simulink subsystem "PowerSystemRef"  (R2024b)
settings: Solver=VariableStepAuto  StartTime=0.0  StopTime=10.0  RelTol=1e-3
undefined symbols (not defined in the file): ess, geom, mot, mot2, mot3, mot4, propel, propel2, propel3, propel4, pxf_diagram_options, SimIn, tc, tc2, tc3, tc4
libraries: simulink x10, slpidlib x5
(part 1 of 10)
settings Model: Creator=drhill  LastModifiedBy=John Clardy
settings SolverCC: AlgebraicLoopSolver=TrustRegion
settings OptimizationCC: ReuseModelBlockBuffer=off
settings DebuggingCC: UnconnectedInputMsg=warning  UnconnectedOutputMsg=warning  UnconnectedLineMsg=warning
settings ModelReferenceCC: EnableRefExpFcnMdlSchedulingChecks=on
settings RTWCC: GPUComputeCapability=3.5  DLArmComputeVersion=19.05

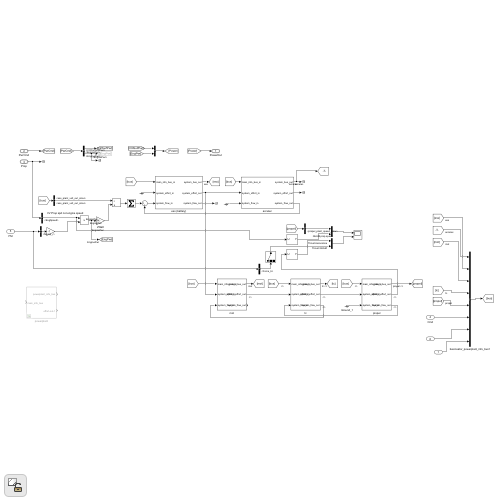
[thumbnail: Simulink's stored preview of the top-level diagram]
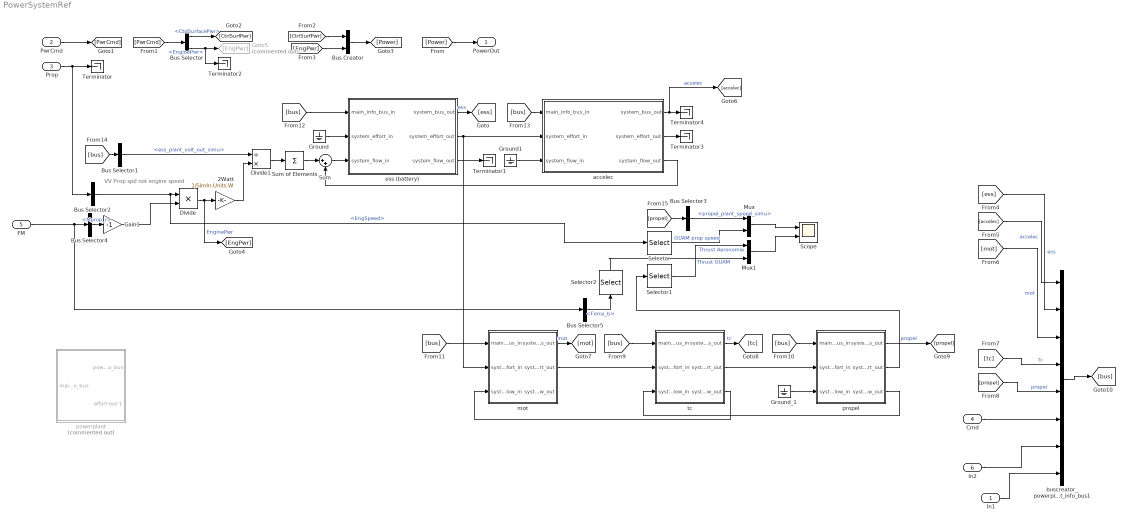
== system PowerSystemRef ==
  note: VV Prop spd not engine speed
  In1 : Inport
  PwrCmd : Inport  Port=2  OutDataTypeStr=Bus: BUS_POWER_SYSTEM_IN
  Prop : Inport  Port=3  OutDataTypeStr=Bus: BUS_PROP_ACTUATOR
  Cmd : Inport  Port=4
  FM : Inport  Port=5
  In2 : Inport  Port=6
  2Watt : Gain  Gain=1/SimIn.Units.W
  Bus Creator : BusCreator  Inputs=2  OutDataTypeStr=Bus: BUS_POWER_SYSTEM_OUT
  Bus Selector : BusSelector  OutputSignals=CtrlSurfacePwr,EnginePwr
  Bus Selector1 : BusSelector  OutputSignals=ess.plant.ess_plant_volt_out_simu
  Bus Selector2 : BusSelector  OutputSignals=EngSpeed
  Bus Selector3 : BusSelector  OutputSignals=propel_plant_speed_simu
  Bus Selector4 : BusSelector  OutputSignals=Propulsion.Mprop_r
  Bus Selector5 : BusSelector  OutputSignals=Propulsion.Force_b
  Divide : Product  Inputs=**
  Divide1 : Product  Inputs=/*
  Gain1 : Gain  Gain=-1
  Goto5 : Goto  Commented=on  GotoTag=EngPwr
  Ground : Ground
  Ground1 : Ground
  Ground_1 : Ground
  Mux : Mux  Inputs=2
  Mux1 : Mux  Inputs=2
  Scope : Scope  NumInputPorts=2
  Selector : Selector  InputPortWidth=9  IndexOptions=Index vector (dialog)  Indices=9  OutputSizes=1
  Selector1 : Selector  InputPortWidth=6  IndexOptions=Index vector (dialog)  Indices=1  OutputSizes=1
  Selector2 : Selector  InputPortWidth=3  IndexOptions=Index vector (dialog)  Indices=1  OutputSizes=1
  Sum : Sum  Inputs=|++
  Sum of Elements : Sum  Inputs=+
  Terminator{,1..4} (5 alike) : Terminator
  accelec : Subsystem
  buscreator_powerplant_info_bus1 : BusCreator  Inputs=8
  ess (battery) : Subsystem
  mot : Subsystem
  powerplant : Subsystem  Commented=on
  propel : Subsystem
  tc : Subsystem
  PowerOut : Outport  OutDataTypeStr=Bus: BUS_POWER_SYSTEM_OUT  VectorParamsAs1DForOutWhenUnconnected=off
  wires:
  Bus Creator/1 -> [Power]
  [Power] -> PowerOut/1
  PwrCmd/1 -> [PwrCmd]
  [PwrCmd] -> Bus Selector/1
  Bus Selector/1 -> [CtrlSurfPwr]  "<CtrlSurfacePwr>"
  [CtrlSurfPwr] -> Bus Creator/1
  [EngPwr] -> Bus Creator/2
  Ground/1 -> ess (battery)/2(system_effort_in)
  Bus Selector2/1 -> Divide/1, Selector/1  "<EngSpeed>"
  Divide1/1 -> Sum of Elements/1
  Prop/1 -> Terminator/1, Bus Selector2/1
  Divide/1 -> 2Watt/1, [EngPwr]  "EnginePwr"
  ess (battery)/3(system_flow_out) -> Terminator1/1
  Bus Selector1/1 -> Divide1/1  "<ess_plant_volt_out_simu>"
  Sum of Elements/1 -> Sum/1
  2Watt/1 -> Divide1/2
  Bus Selector4/1 -> Gain1/1  "<Mprop_r>"
  FM/1 -> Bus Selector4/1, Bus Selector5/1
  Gain1/1 -> Divide/2
  Bus Selector/2 -> Goto5/1, Terminator2/1  "<EnginePwr>"
  ess (battery)/2(system_effort_out) -> mot/2(system_effort_in), accelec/2(system_effort_in)
  Ground1/1 -> accelec/3(system_flow_in)
  Sum/1 -> ess (battery)/3(system_flow_in)
  accelec/3(system_flow_out) -> Sum/2
  accelec/2(system_effort_out) -> Terminator3/1
  accelec/1(system_bus_out) -> Terminator4/1, [accelec]  "accelec"
  [accelec] -> buscreator_powerplant_info_bus1/1  "accelec"
  [ess] -> buscreator_powerplant_info_bus1/2  "ess"
  [mot] -> buscreator_powerplant_info_bus1/3  "mot"
  mot/1(system_bus_out) -> [mot]  "mot"
  [tc] -> buscreator_powerplant_info_bus1/4  "tc"
  [propel] -> buscreator_powerplant_info_bus1/5  "propel"
  buscreator_powerplant_info_bus1/1 -> [bus]
  [bus] -> mot/1(main_info_bus_in)
  Cmd/1 -> buscreator_powerplant_info_bus1/6
  In1/1 -> buscreator_powerplant_info_bus1/8
  [bus] -> ess (battery)/1(main_info_bus_in)
  [bus] -> accelec/1(main_info_bus_in)
  ess (battery)/1(system_bus_out) -> [ess]  "ess"
  [bus] -> Bus Selector1/1
  In2/1 -> buscreator_powerplant_info_bus1/7
  Mux/1 -> Scope/1
  Mux1/1 -> Scope/2
  [propel] -> Bus Selector3/1
  Bus Selector3/1 -> Mux/1  "<propel_plant_speed_simu>"
  Selector/1 -> Mux/2  "GUAM prop speed"
  Selector1/1 -> Mux1/1  "Thrust Aeronomie"
  Bus Selector5/1 -> Selector2/1  "<Force_b>"
  Selector2/1 -> Mux1/2  "Thrust GUAM"
  mot/2(system_effort_out) -> tc/2(system_effort_in)
  tc/3(system_flow_out) -> mot/3(system_flow_in)
  tc/1(system_bus_out) -> [tc]  "tc"
  [bus] -> tc/1(main_info_bus_in)
  propel/2(system_effort_out) -> Selector1/1
  Ground_1/1 -> propel/3(system_flow_in)
  tc/2(system_effort_out) -> propel/2(system_effort_in)
  propel/3(system_flow_out) -> tc/3(system_flow_in)
  [bus] -> propel/1(main_info_bus_in)
  propel/1(system_bus_out) -> [propel]  "propel"

== system PowerSystemRef/accelec ==
  main_info_bus_in : Inport
  system_effort_in : Inport  Port=2
  system_flow_in : Inport  Port=3
  Ground_1 : Ground
  Terminator_1 : Terminator
  plant : Subsystem
      mask Display: disp('accelec_plant_const_pwrloss_volt_in_nokey.slx')
  system_bus_out : Outport
  system_effort_out : Outport  Port=2
  system_flow_out : Outport  Port=3
  wires:
  main_info_bus_in/1 -> plant/1(aInport--1)
  plant/1(outport-system_info_bus) -> [plant]
  plant/3(out-effort-6) -> system_effort_out/1
  plant/4(out-flow-7) -> system_flow_out/1
  system_effort_in/1 -> plant/3(in-effort-2)
  system_flow_in/1 -> plant/4(in-flow-3)
  [plant] -> system_bus_out/1  "plant"
  Ground_1/1 -> plant/2(aInport--2)
  plant/2(aOutport--2) -> Terminator_1/1

== system PowerSystemRef/ess (battery) ==
  main_info_bus_in : Inport
  system_effort_in : Inport  Port=2
  system_flow_in : Inport  Port=3
  buscreator_system_bus_out1 : BusCreator  Inputs=2
  ctrl : Subsystem
      mask Display: disp('ess_ctrl_pngv_map_anl_PI_cstr.slx')
  memoryctrl : Memory
  plant : Subsystem
      mask Display: disp('ess_plant_pngv_map_anl_PI_cstr.slx')
  system_bus_out : Outport
  system_effort_out : Outport  Port=2
  system_flow_out : Outport  Port=3
  wires:
  ctrl/1(outport-system_info_bus) -> [ctrl]  "system_info_bus"
  ctrl/2(outport-ctrl_bus) -> memoryctrl/1  "ctrl_bus"
  main_info_bus_in/1 -> ctrl/1(inport-main_info_bus-1), plant/1(aInport--1)  "main_info_bus"
  plant/2(outport-plant_bus) -> ctrl/2(aInport--2)  "plant_bus"
  memoryctrl/1 -> plant/2(aInport--2)  "ctrl_bus"
  plant/1(outport-system_info_bus) -> [plant]  "system_info_bus"
  plant/3(out-effort-12) -> system_effort_out/1  "effort"
  plant/4(out-flow-13) -> system_flow_out/1  "flow"
  system_effort_in/1 -> plant/3(in-effort-1)  "effort"
  system_flow_in/1 -> plant/4(in-flow-2)  "flow"
  buscreator_system_bus_out1/1 -> system_bus_out/1  "system_info_bus"
  [ctrl] -> buscreator_system_bus_out1/1  "ctrl"
  [plant] -> buscreator_system_bus_out1/2  "plant"

== system PowerSystemRef/mot ==
  main_info_bus_in : Inport
  system_effort_in : Inport  Port=2
  system_flow_in : Inport  Port=3
  buscreator_system_bus_out1 : BusCreator  Inputs=2
  ctrl : Subsystem
  memoryctrl : Memory
  plant : Subsystem
      mask Display: disp('mot_plant_map_Pelec_funTW_volt_in.slx')
  system_bus_out : Outport
  system_effort_out : Outport  Port=2
  system_flow_out : Outport  Port=3
  wires:
  ctrl/1(system_bus_out) -> [ctrl]  "system_info_bus"
  ctrl/2(local_info_bus_out) -> memoryctrl/1  "ctrl_bus"
  main_info_bus_in/1 -> ctrl/1(main_info_bus_in), plant/1(aInport--1)  "main_info_bus"
  plant/2(outport-plant_bus) -> ctrl/2(local_info_bus_in)  "plant_bus"
  memoryctrl/1 -> plant/2(inport-ctrl_bus-2)  "ctrl_bus"
  plant/1(outport-system_info_bus) -> [plant]  "system_info_bus"
  plant/3(out-effort-7) -> system_effort_out/1  "effort"
  plant/4(out-flow-8) -> system_flow_out/1  "flow"
  system_effort_in/1 -> plant/3(in-effort-2)  "effort"
  system_flow_in/1 -> plant/4(in-flow-3)  "flow"
  buscreator_system_bus_out1/1 -> system_bus_out/1  "system_info_bus"
  [ctrl] -> buscreator_system_bus_out1/1  "ctrl"
  [plant] -> buscreator_system_bus_out1/2  "plant"

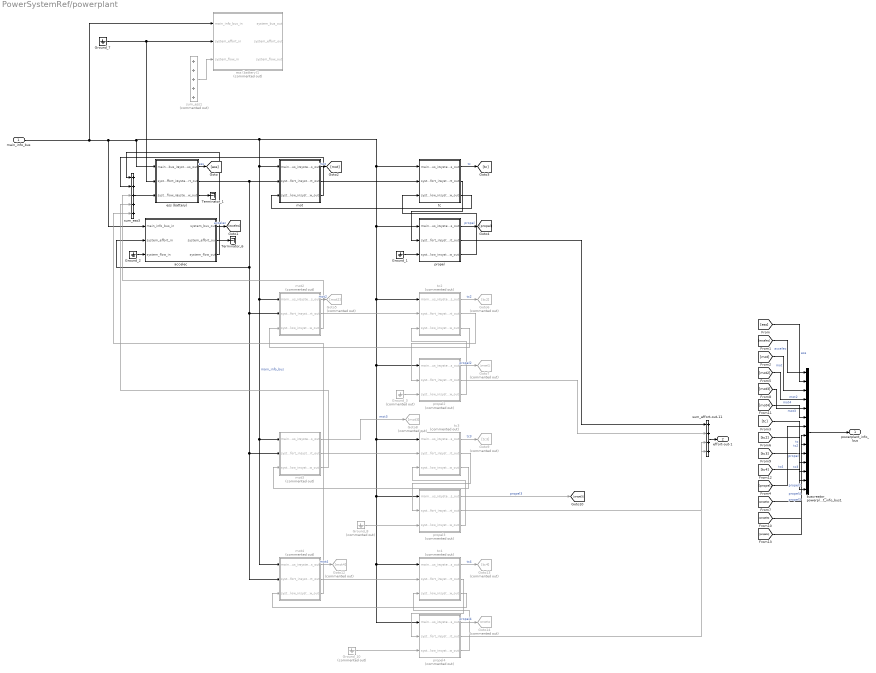
== system PowerSystemRef/powerplant ==
  main_info_bus : Inport
  Goto12 : Goto  Commented=on  GotoTag=mot4
  Goto13 : Goto  Commented=on  GotoTag=tc4
  Goto14 : Goto  Commented=on  GotoTag=propel4
  Goto5 : Goto  Commented=on  GotoTag=mot2
  Goto6 : Goto  Commented=on  GotoTag=tc2
  Goto7 : Goto  Commented=on  GotoTag=propel2
  Goto8 : Goto  Commented=on  GotoTag=mot3
  Goto9 : Goto  Commented=on  GotoTag=tc3
  Ground_1 : Ground
  Ground_10 : Ground  Commented=on
  Ground_2 : Ground
  Ground_3 : Ground  Commented=on
  Ground_7 : Ground
  Ground_8 : Ground  Commented=on
  Terminator_1 : Terminator
  Terminator_6 : Terminator
  accelec : Subsystem
  buscreator_powerplant_info_bus1 : BusCreator  Inputs=14
  ess (battery) : Subsystem
  ess (battery)1 : Subsystem  Commented=on
  mot : Subsystem
  mot2 : Subsystem  Commented=on
  mot3 : Subsystem  Commented=on
  mot4 : Subsystem  Commented=on
  propel : Subsystem
  propel2 : Subsystem  Commented=on
  propel3 : Subsystem  Commented=on
  propel4 : Subsystem  Commented=on
  sum_effort-out-11 : Sum  Inputs=++++
  sum_ess1 : Sum  Commented=on  Inputs=+++++
  sum_ess3 : Sum  Inputs=+++++
  tc : Subsystem
  tc2 : Subsystem  Commented=on
  tc3 : Subsystem  Commented=on
  tc4 : Subsystem  Commented=on
  powerplant_info_bus : Outport  VectorParamsAs1DForOutWhenUnconnected=off
  effort-out-1 : Outport  Port=2  VectorParamsAs1DForOutWhenUnconnected=off
  wires:
  Ground_2/1 -> accelec/3(system_flow_in)
  accelec/1(system_bus_out) -> [accelec]  "accelec"
  accelec/2(system_effort_out) -> Terminator_6/1
  accelec/3(system_flow_out) -> sum_ess3/1
  ess (battery)/2(system_effort_out) -> mot3/2(system_effort_in), mot4/2(system_effort_in), mot2/2(system_effort_in), accelec/2(system_effort_in), mot/2(system_effort_in)
  main_info_bus/1 -> mot3/1(main_info_bus_in), mot4/1(main_info_bus_in), mot2/1(main_info_bus_in), mot/1(main_info_bus_in), propel4/1(main_info_bus_in), tc4/1(main_info_bus_in), propel3/1(main_info_bus_in), tc3/1(main_info_bus_in), propel2/1(main_info_bus_in), tc2/1(main_info_bus_in), propel/1(main_info_bus_in), tc/1(main_info_bus_in), ess (battery)/1(main_info_bus_in), accelec/1(main_info_bus_in), ess (battery)1/1(main_info_bus_in)  "main_info_bus"
  Ground_7/1 -> ess (battery)/2(system_effort_in), ess (battery)1/2(system_effort_in)
  ess (battery)/1(system_bus_out) -> [ess]  "ess"
  ess (battery)/3(system_flow_out) -> Terminator_1/1
  sum_ess3/1 -> ess (battery)/3(system_flow_in)
  mot/1(system_bus_out) -> [mot]  "mot"
  mot/2(system_effort_out) -> tc/2(system_effort_in)
  mot/3(system_flow_out) -> sum_ess3/2
  tc/3(system_flow_out) -> mot/3(system_flow_in)
  mot2/1(system_bus_out) -> Goto5/1  "mot2"
  mot2/2(system_effort_out) -> tc2/2(system_effort_in)
  mot2/3(system_flow_out) -> sum_ess3/3
  tc2/3(system_flow_out) -> mot2/3(system_flow_in)
  mot3/1(system_bus_out) -> Goto8/1  "mot3"
  mot3/2(system_effort_out) -> tc3/2(system_effort_in)
  mot3/3(system_flow_out) -> sum_ess3/4
  tc3/3(system_flow_out) -> mot3/3(system_flow_in)
  mot4/1(system_bus_out) -> Goto12/1  "mot4"
  mot4/2(system_effort_out) -> tc4/2(system_effort_in)
  mot4/3(system_flow_out) -> sum_ess3/5
  tc4/3(system_flow_out) -> mot4/3(system_flow_in)
  Ground_1/1 -> propel/3(system_flow_in)
  propel/1(system_bus_out) -> [propel]  "propel"
  propel/2(system_effort_out) -> sum_effort-out-11/1
  propel/3(system_flow_out) -> tc/3(system_flow_in)
  tc/2(system_effort_out) -> propel/2(system_effort_in)
  Ground_3/1 -> propel2/3(system_flow_in)
  propel2/1(system_bus_out) -> Goto7/1  "propel2"
  propel2/2(system_effort_out) -> sum_effort-out-11/2
  propel2/3(system_flow_out) -> tc2/3(system_flow_in)
  tc2/2(system_effort_out) -> propel2/2(system_effort_in)
  Ground_8/1 -> propel3/3(system_flow_in)
  propel3/1(system_bus_out) -> [propel3]  "propel3"
  propel3/2(system_effort_out) -> sum_effort-out-11/3
  propel3/3(system_flow_out) -> tc3/3(system_flow_in)
  tc3/2(system_effort_out) -> propel3/2(system_effort_in)
  Ground_10/1 -> propel4/3(system_flow_in)
  propel4/1(system_bus_out) -> Goto14/1  "propel4"
  propel4/2(system_effort_out) -> sum_effort-out-11/4
  propel4/3(system_flow_out) -> tc4/3(system_flow_in)
  tc4/2(system_effort_out) -> propel4/2(system_effort_in)
  tc/1(system_bus_out) -> [tc]  "tc"
  tc2/1(system_bus_out) -> Goto6/1  "tc2"
  tc3/1(system_bus_out) -> Goto9/1  "tc3"
  tc4/1(system_bus_out) -> Goto13/1  "tc4"
  buscreator_powerplant_info_bus1/1 -> powerplant_info_bus/1
  sum_effort-out-11/1 -> effort-out-1/1
  [accelec] -> buscreator_powerplant_info_bus1/1  "accelec"
  [ess] -> buscreator_powerplant_info_bus1/2  "ess"
  [mot] -> buscreator_powerplant_info_bus1/3  "mot"
  [mot2] -> buscreator_powerplant_info_bus1/4  "mot2"
  [mot3] -> buscreator_powerplant_info_bus1/5  "mot3"
  [mot4] -> buscreator_powerplant_info_bus1/6  "mot4"
  [propel] -> buscreator_powerplant_info_bus1/7  "propel"
  [propel2] -> buscreator_powerplant_info_bus1/8  "propel2"
  [propel3] -> buscreator_powerplant_info_bus1/9  "propel3"
  [propel4] -> buscreator_powerplant_info_bus1/10  "propel4"
  [tc] -> buscreator_powerplant_info_bus1/11  "tc"
  [tc2] -> buscreator_powerplant_info_bus1/12  "tc2"
  [tc3] -> buscreator_powerplant_info_bus1/13  "tc3"
  [tc4] -> buscreator_powerplant_info_bus1/14  "tc4"
  sum_ess1/1 -> ess (battery)1/3(system_flow_in)

== system PowerSystemRef/propel ==
  main_info_bus_in : Inport
  system_effort_in : Inport  Port=2
  system_flow_in : Inport  Port=3
  Ground_1 : Ground
  Terminator_1 : Terminator
  plant : Subsystem
      mask Display: disp('propel_plant_uas.slx')
  system_bus_out : Outport
  system_effort_out : Outport  Port=2
  system_flow_out : Outport  Port=3
  wires:
  main_info_bus_in/1 -> plant/1(inport-main_info_bus-1)
  plant/1(outport-system_info_bus) -> [plant]
  plant/3(out-effort-5) -> system_effort_out/1
  plant/4(out-flow-6) -> system_flow_out/1
  system_effort_in/1 -> plant/3(in-effort-4)
  system_flow_in/1 -> plant/4(in-flow-5)
  [plant] -> system_bus_out/1  "plant"
  Ground_1/1 -> plant/2(aInport--2)
  plant/2(aOutport--2) -> Terminator_1/1

== system PowerSystemRef/tc ==
  main_info_bus_in : Inport
  system_effort_in : Inport  Port=2
  system_flow_in : Inport  Port=3
  Ground_1 : Ground
  Terminator_1 : Terminator
  plant : Subsystem
      mask Display: disp('tc_plant_map_trqloss_funTW.slx')
  system_bus_out : Outport
  system_effort_out : Outport  Port=2
  system_flow_out : Outport  Port=3
  wires:
  main_info_bus_in/1 -> plant/1(aInport--1)
  plant/1(outport-system_info_bus) -> [plant]
  plant/3(out-effort-7) -> system_effort_out/1
  plant/4(out-flow-8) -> system_flow_out/1
  system_effort_in/1 -> plant/3(in-effort-1)
  system_flow_in/1 -> plant/4(in-flow-2)
  [plant] -> system_bus_out/1  "plant"
  Ground_1/1 -> plant/2(aInport--2)
  plant/2(aOutport--2) -> Terminator_1/1

== system PowerSystemRef/accelec/plant ==
  aInport--1 : Inport
  aInport--2 : Inport  Port=2
  in-effort-2 : Inport  Port=3
  in-flow-3 : Inport  Port=4
  Ground_1 : Ground
  Ground_2 : Ground
  Terminator_1 : Terminator
  Terminator_2 : Terminator
  accelec_plant_const_pwrloss_volt_in_nokey : Subsystem
  parameter_out : Subsystem
  parameter_selection : Subsystem
  outport-system_info_bus : Outport
  aOutport--2 : Outport  Port=2
  out-effort-6 : Outport  Port=3
  out-flow-7 : Outport  Port=4
  wires:
  parameter_out/1(outport-system_info_bus) -> outport-system_info_bus/1
  accelec_plant_const_pwrloss_volt_in_nokey/1(accelec_plant_volt_in_simu) -> parameter_out/1(inport-accelec_plant_volt_in_simu)
  accelec_plant_const_pwrloss_volt_in_nokey/2(accelec_plant_pwr_simu) -> parameter_out/2(inport-accelec_plant_pwr_simu)
  accelec_plant_const_pwrloss_volt_in_nokey/3(accelec_plant_curr_in_simu) -> parameter_out/3(inport-accelec_plant_curr_in_simu)
  accelec_plant_const_pwrloss_volt_in_nokey/4(accelec_plant_volt_out_simu) -> parameter_out/4(inport-accelec_plant_volt_out_simu)
  accelec_plant_const_pwrloss_volt_in_nokey/5(accelec_plant_curr_out_simu) -> parameter_out/5(inport-accelec_plant_curr_out_simu)
  in-effort-2/1 -> accelec_plant_const_pwrloss_volt_in_nokey/2(accelec_volt_in)
  in-flow-3/1 -> accelec_plant_const_pwrloss_volt_in_nokey/3(accelec_curr_out)
  accelec_plant_const_pwrloss_volt_in_nokey/6(accelec_volt_out) -> out-effort-6/1
  accelec_plant_const_pwrloss_volt_in_nokey/7(accelec_curr_in) -> out-flow-7/1
  aInport--1/1 -> Terminator_1/1
  aInport--2/1 -> Terminator_2/1
  Ground_1/1 -> accelec_plant_const_pwrloss_volt_in_nokey/1(drv_key_on_dmd_simu)
  Ground_2/1 -> aOutport--2/1

== system PowerSystemRef/ess (battery)/ctrl ==
  inport-main_info_bus-1 : Inport
  aInport--2 : Inport  Port=2
  Terminator_1 : Terminator
  ess_ctrl_pngv_map_anl_PI_cstr : Subsystem
  parameter_out : Subsystem
  parameter_selection : Subsystem
  outport-system_info_bus : Outport
  outport-ctrl_bus : Outport  Port=2
  wires:
  inport-main_info_bus-1/1 -> parameter_selection/1(inport-main_info_bus-1)
  parameter_out/1(outport-system_info_bus) -> outport-system_info_bus/1
  parameter_out/2(outport-ctrl_bus) -> outport-ctrl_bus/1
  ess_ctrl_pngv_map_anl_PI_cstr/1(ess_ctrl_pwr_max_pro_simu) -> parameter_out/1(inport-ess_ctrl_pwr_max_pro_simu)
  ess_ctrl_pngv_map_anl_PI_cstr/2(ess_ctrl_pwr_max_reg_simu) -> parameter_out/2(inport-ess_ctrl_pwr_max_reg_simu)
  ess_ctrl_pngv_map_anl_PI_cstr/3(ess_ctrl_curr_max_pro_simu) -> parameter_out/3(inport-ess_ctrl_curr_max_pro_simu)
  ess_ctrl_pngv_map_anl_PI_cstr/4(ess_ctrl_curr_max_reg_simu) -> parameter_out/4(inport-ess_ctrl_curr_max_reg_simu)
  parameter_selection/1(outport-ess_plant_volt_out_simu-1) -> ess_ctrl_pngv_map_anl_PI_cstr/1(ess_volt_out)
  parameter_selection/2(outport-ess_plant_curr_out_simu-2) -> ess_ctrl_pngv_map_anl_PI_cstr/2(ess_curr_out)
  parameter_selection/3(outport-ess_plant_soc_simu-3) -> ess_ctrl_pngv_map_anl_PI_cstr/3(ess_soc)
  aInport--2/1 -> Terminator_1/1

== system PowerSystemRef/ess (battery)/plant ==
  aInport--1 : Inport
  aInport--2 : Inport  Port=2
  in-effort-1 : Inport  Port=3
  in-flow-2 : Inport  Port=4
  Terminator_1 : Terminator
  Terminator_2 : Terminator
  ess_plant_pngv_map_anl_PI_cstr : Subsystem
  parameter_out : Subsystem
  parameter_selection : Subsystem
  outport-system_info_bus : Outport
  outport-plant_bus : Outport  Port=2
  out-effort-12 : Outport  Port=3
  out-flow-13 : Outport  Port=4
  wires:
  parameter_out/1(outport-system_info_bus) -> outport-system_info_bus/1
  parameter_out/2(outport-plant_bus) -> outport-plant_bus/1
  ess_plant_pngv_map_anl_PI_cstr/1(ess_plant_soc_simu) -> parameter_out/1(inport-ess_plant_soc_simu)
  ess_plant_pngv_map_anl_PI_cstr/10(ess_plant_heat_out_simu) -> parameter_out/10(inport-ess_plant_heat_out_simu)
  ess_plant_pngv_map_anl_PI_cstr/11(ess_plant_impedance_simu) -> parameter_out/11(inport-ess_plant_impedance_simu)
  ess_plant_pngv_map_anl_PI_cstr/2(ess_plant_curr_out_simu) -> parameter_out/2(inport-ess_plant_curr_out_simu)
  ess_plant_pngv_map_anl_PI_cstr/3(ess_plant_volt_out_simu) -> parameter_out/3(inport-ess_plant_volt_out_simu)
  ess_plant_pngv_map_anl_PI_cstr/4(ess_plant_voc_simu) -> parameter_out/4(inport-ess_plant_voc_simu)
  ess_plant_pngv_map_anl_PI_cstr/5(ess_plant_rint_simu) -> parameter_out/5(inport-ess_plant_rint_simu)
  ess_plant_pngv_map_anl_PI_cstr/6(ess_plant_rpol1_simu) -> parameter_out/6(inport-ess_plant_rpol1_simu)
  ess_plant_pngv_map_anl_PI_cstr/7(ess_plant_rpol2_simu) -> parameter_out/7(inport-ess_plant_rpol2_simu)
  ess_plant_pngv_map_anl_PI_cstr/8(ess_plant_curr_pol1_simu) -> parameter_out/8(inport-ess_plant_curr_pol1_simu)
  ess_plant_pngv_map_anl_PI_cstr/9(ess_plant_curr_pol2_simu) -> parameter_out/9(inport-ess_plant_curr_pol2_simu)
  in-effort-1/1 -> ess_plant_pngv_map_anl_PI_cstr/1(ess_volt_in)
  in-flow-2/1 -> ess_plant_pngv_map_anl_PI_cstr/2(ess_curr_out)
  ess_plant_pngv_map_anl_PI_cstr/12(ess_volt_out) -> out-effort-12/1
  ess_plant_pngv_map_anl_PI_cstr/13(ess_curr_in) -> out-flow-13/1
  aInport--1/1 -> Terminator_1/1
  aInport--2/1 -> Terminator_2/1

== system PowerSystemRef/mot/ctrl ==
  main_info_bus_in : Inport
  local_info_bus_in : Inport  Port=2
  buscreator_system_bus_out1 : BusCreator  Inputs=3
  cmd : Subsystem
      mask Display: disp('mot_ctrl_cmd_map_Pelec_funTW_volt_in.slx')
  cstr : Subsystem
      mask Display: disp('mot_ctrl_cstr_map_Pelec_funTW_volt_in.slx')
  dmd : Subsystem
      mask Display: disp('mot_ctrl_dmd_uas.slx')
  system_bus_out : Outport
  local_info_bus_out : Outport  Port=2
  wires:
  dmd/1(outport-system_info_bus) -> [dmd]
  dmd/2(outport-dmd_bus) -> cmd/4(aInport--4), cstr/3(aInport--3)
  [local_info_bus] -> dmd/2(aInport--2)
  [main_info_bus] -> dmd/1(inport-main_info_bus-1)
  cstr/1(outport-system_info_bus) -> [cstr]
  cstr/2(outport-cstr_bus) -> cmd/3(aInport--3)
  [local_info_bus] -> cstr/2(aInport--2)
  [main_info_bus] -> cstr/1(inport-main_info_bus-1)
  cmd/1(outport-system_info_bus) -> local_info_bus_out/1, [cmd]
  [local_info_bus] -> cmd/2(aInport--2)
  [main_info_bus] -> cmd/1(inport-main_info_bus-1)
  main_info_bus_in/1 -> [main_info_bus]
  local_info_bus_in/1 -> [local_info_bus]
  buscreator_system_bus_out1/1 -> system_bus_out/1
  [cmd] -> buscreator_system_bus_out1/1  "cmd"
  [cstr] -> buscreator_system_bus_out1/2  "cstr"
  [dmd] -> buscreator_system_bus_out1/3  "dmd"

== system PowerSystemRef/mot/plant ==
  aInport--1 : Inport
  inport-ctrl_bus-2 : Inport  Port=2
  in-effort-2 : Inport  Port=3
  in-flow-3 : Inport  Port=4
  Ground_1 : Ground
  Terminator_1 : Terminator
  mot_plant_map_Pelec_funTW_volt_in : Subsystem
  parameter_out : Subsystem
  parameter_selection : Subsystem
  outport-system_info_bus : Outport
  outport-plant_bus : Outport  Port=2
  out-effort-7 : Outport  Port=3
  out-flow-8 : Outport  Port=4
  wires:
  inport-ctrl_bus-2/1 -> parameter_selection/2(inport-ctrl_bus-2)
  parameter_out/1(outport-system_info_bus) -> outport-system_info_bus/1
  parameter_out/2(outport-plant_bus) -> outport-plant_bus/1
  mot_plant_map_Pelec_funTW_volt_in/1(mot_plant_spd_out_simu) -> parameter_out/1(inport-mot_plant_spd_out_simu)
  mot_plant_map_Pelec_funTW_volt_in/2(mot_plant_curr_in_simu) -> parameter_out/2(inport-mot_plant_curr_in_simu)
  mot_plant_map_Pelec_funTW_volt_in/3(mot_plant_volt_in_simu) -> parameter_out/3(inport-mot_plant_volt_in_simu)
  mot_plant_map_Pelec_funTW_volt_in/4(mot_plant_cmd_simu) -> parameter_out/4(inport-mot_plant_cmd_simu)
  mot_plant_map_Pelec_funTW_volt_in/5(mot_plant_trq_out_simu) -> parameter_out/5(inport-mot_plant_trq_out_simu)
  mot_plant_map_Pelec_funTW_volt_in/6(mot_plant_temp_coeff_simu) -> parameter_out/6(inport-mot_plant_temp_coeff_simu)
  parameter_selection/1(outport-mot_ctrl_cmd_simu-1) -> mot_plant_map_Pelec_funTW_volt_in/1(mot_ctrl_cmd_simu)
  in-effort-2/1 -> mot_plant_map_Pelec_funTW_volt_in/2(voltage)
  in-flow-3/1 -> mot_plant_map_Pelec_funTW_volt_in/3(spd)
  mot_plant_map_Pelec_funTW_volt_in/7(mot_trq_out mot_inertia_out) -> out-effort-7/1
  mot_plant_map_Pelec_funTW_volt_in/8(mot_current_out) -> out-flow-8/1
  aInport--1/1 -> Terminator_1/1
  Ground_1/1 -> parameter_selection/1(Inport_1)

== system PowerSystemRef/powerplant/accelec ==
  main_info_bus_in : Inport
  system_effort_in : Inport  Port=2
  system_flow_in : Inport  Port=3
  Ground_1 : Ground
  Terminator_1 : Terminator
  plant : Subsystem
      mask Display: disp('accelec_plant_const_pwrloss_volt_in_nokey.slx')
  system_bus_out : Outport
  system_effort_out : Outport  Port=2
  system_flow_out : Outport  Port=3
  wires:
  main_info_bus_in/1 -> plant/1(aInport--1)
  plant/1(outport-system_info_bus) -> [plant]
  plant/3(out-effort-6) -> system_effort_out/1
  plant/4(out-flow-7) -> system_flow_out/1
  system_effort_in/1 -> plant/3(in-effort-2)
  system_flow_in/1 -> plant/4(in-flow-3)
  [plant] -> system_bus_out/1  "plant"
  Ground_1/1 -> plant/2(aInport--2)
  plant/2(aOutport--2) -> Terminator_1/1

== system PowerSystemRef/powerplant/ess (battery) ==
  main_info_bus_in : Inport
  system_effort_in : Inport  Port=2
  system_flow_in : Inport  Port=3
  buscreator_system_bus_out1 : BusCreator  Inputs=2
  ctrl : Subsystem
      mask Display: disp('ess_ctrl_pngv_map_anl_PI_cstr.slx')
  memoryctrl : Memory
  plant : Subsystem
      mask Display: disp('ess_plant_pngv_map_anl_PI_cstr.slx')
  system_bus_out : Outport
  system_effort_out : Outport  Port=2
  system_flow_out : Outport  Port=3
  wires:
  ctrl/1(outport-system_info_bus) -> [ctrl]  "system_info_bus"
  ctrl/2(outport-ctrl_bus) -> memoryctrl/1  "ctrl_bus"
  main_info_bus_in/1 -> ctrl/1(inport-main_info_bus-1), plant/1(aInport--1)  "main_info_bus"
  plant/2(outport-plant_bus) -> ctrl/2(aInport--2)  "plant_bus"
  memoryctrl/1 -> plant/2(aInport--2)  "ctrl_bus"
  plant/1(outport-system_info_bus) -> [plant]  "system_info_bus"
  plant/3(out-effort-12) -> system_effort_out/1  "effort"
  plant/4(out-flow-13) -> system_flow_out/1  "flow"
  system_effort_in/1 -> plant/3(in-effort-1)  "effort"
  system_flow_in/1 -> plant/4(in-flow-2)  "flow"
  buscreator_system_bus_out1/1 -> system_bus_out/1  "system_info_bus"
  [ctrl] -> buscreator_system_bus_out1/1  "ctrl"
  [plant] -> buscreator_system_bus_out1/2  "plant"

== system PowerSystemRef/powerplant/ess (battery)1 ==
  main_info_bus_in : Inport
  system_effort_in : Inport  Port=2
  system_flow_in : Inport  Port=3
  buscreator_system_bus_out1 : BusCreator  Inputs=2
  ctrl : Subsystem
      mask Display: disp('ess_ctrl_pngv_map_anl_PI_cstr.slx')
  memoryctrl : Memory
  plant : Subsystem
      mask Display: disp('ess_plant_pngv_map_anl_PI_cstr.slx')
  system_bus_out : Outport
  system_effort_out : Outport  Port=2
  system_flow_out : Outport  Port=3
  wires:
  [plant] -> buscreator_system_bus_out1/2  "plant"
  [ctrl] -> buscreator_system_bus_out1/1  "ctrl"
  buscreator_system_bus_out1/1 -> system_bus_out/1  "system_info_bus"
  system_flow_in/1 -> plant/4(in-flow-2)  "flow"
  system_effort_in/1 -> plant/3(in-effort-1)  "effort"
  plant/4(out-flow-13) -> system_flow_out/1  "flow"
  plant/3(out-effort-12) -> system_effort_out/1  "effort"
  plant/1(outport-system_info_bus) -> [plant]  "system_info_bus"
  memoryctrl/1 -> plant/2(aInport--2)  "ctrl_bus"
  plant/2(outport-plant_bus) -> ctrl/2(aInport--2)  "plant_bus"
  main_info_bus_in/1 -> plant/1(aInport--1), ctrl/1(inport-main_info_bus-1)  "main_info_bus"
  ctrl/2(outport-ctrl_bus) -> memoryctrl/1  "ctrl_bus"
  ctrl/1(outport-system_info_bus) -> [ctrl]  "system_info_bus"

== system PowerSystemRef/powerplant/mot ==
  main_info_bus_in : Inport
  system_effort_in : Inport  Port=2
  system_flow_in : Inport  Port=3
  buscreator_system_bus_out1 : BusCreator  Inputs=2
  ctrl : Subsystem
  memoryctrl : Memory
  plant : Subsystem
      mask Display: disp('mot_plant_map_Pelec_funTW_volt_in.slx')
  system_bus_out : Outport
  system_effort_out : Outport  Port=2
  system_flow_out : Outport  Port=3
  wires:
  ctrl/1(system_bus_out) -> [ctrl]  "system_info_bus"
  ctrl/2(local_info_bus_out) -> memoryctrl/1  "ctrl_bus"
  main_info_bus_in/1 -> ctrl/1(main_info_bus_in), plant/1(aInport--1)  "main_info_bus"
  plant/2(outport-plant_bus) -> ctrl/2(local_info_bus_in)  "plant_bus"
  memoryctrl/1 -> plant/2(inport-ctrl_bus-2)  "ctrl_bus"
  plant/1(outport-system_info_bus) -> [plant]  "system_info_bus"
  plant/3(out-effort-7) -> system_effort_out/1  "effort"
  plant/4(out-flow-8) -> system_flow_out/1  "flow"
  system_effort_in/1 -> plant/3(in-effort-2)  "effort"
  system_flow_in/1 -> plant/4(in-flow-3)  "flow"
  buscreator_system_bus_out1/1 -> system_bus_out/1  "system_info_bus"
  [ctrl] -> buscreator_system_bus_out1/1  "ctrl"
  [plant] -> buscreator_system_bus_out1/2  "plant"

== system PowerSystemRef/powerplant/mot2 ==
  main_info_bus_in : Inport
  system_effort_in : Inport  Port=2
  system_flow_in : Inport  Port=3
  buscreator_system_bus_out1 : BusCreator  Inputs=2
  ctrl : Subsystem
  memoryctrl : Memory
  plant : Subsystem
      mask Display: disp('mot2_plant_map_Pelec_funTW_volt_in.slx')
  system_bus_out : Outport
  system_effort_out : Outport  Port=2
  system_flow_out : Outport  Port=3
  wires:
  ctrl/1(system_bus_out) -> [ctrl]  "system_info_bus"
  ctrl/2(local_info_bus_out) -> memoryctrl/1  "ctrl_bus"
  main_info_bus_in/1 -> ctrl/1(main_info_bus_in), plant/1(aInport--1)  "main_info_bus"
  plant/2(outport-plant_bus) -> ctrl/2(local_info_bus_in)  "plant_bus"
  memoryctrl/1 -> plant/2(inport-ctrl_bus-2)  "ctrl_bus"
  plant/1(outport-system_info_bus) -> [plant]  "system_info_bus"
  plant/3(out-effort-7) -> system_effort_out/1  "effort"
  plant/4(out-flow-8) -> system_flow_out/1  "flow"
  system_effort_in/1 -> plant/3(in-effort-2)  "effort"
  system_flow_in/1 -> plant/4(in-flow-3)  "flow"
  buscreator_system_bus_out1/1 -> system_bus_out/1  "system_info_bus"
  [ctrl] -> buscreator_system_bus_out1/1  "ctrl"
  [plant] -> buscreator_system_bus_out1/2  "plant"

== system PowerSystemRef/powerplant/mot3 ==
  main_info_bus_in : Inport
  system_effort_in : Inport  Port=2
  system_flow_in : Inport  Port=3
  buscreator_system_bus_out1 : BusCreator  Inputs=2
  ctrl : Subsystem
  memoryctrl : Memory
  plant : Subsystem
      mask Display: disp('mot3_plant_map_Pelec_funTW_volt_in.slx')
  system_bus_out : Outport
  system_effort_out : Outport  Port=2
  system_flow_out : Outport  Port=3
  wires:
  ctrl/1(system_bus_out) -> [ctrl]  "system_info_bus"
  ctrl/2(local_info_bus_out) -> memoryctrl/1  "ctrl_bus"
  main_info_bus_in/1 -> ctrl/1(main_info_bus_in), plant/1(aInport--1)  "main_info_bus"
  plant/2(outport-plant_bus) -> ctrl/2(local_info_bus_in)  "plant_bus"
  memoryctrl/1 -> plant/2(inport-ctrl_bus-2)  "ctrl_bus"
  plant/1(outport-system_info_bus) -> [plant]  "system_info_bus"
  plant/3(out-effort-7) -> system_effort_out/1  "effort"
  plant/4(out-flow-8) -> system_flow_out/1  "flow"
  system_effort_in/1 -> plant/3(in-effort-2)  "effort"
  system_flow_in/1 -> plant/4(in-flow-3)  "flow"
  buscreator_system_bus_out1/1 -> system_bus_out/1  "system_info_bus"
  [ctrl] -> buscreator_system_bus_out1/1  "ctrl"
  [plant] -> buscreator_system_bus_out1/2  "plant"

== system PowerSystemRef/powerplant/mot4 ==
  main_info_bus_in : Inport
  system_effort_in : Inport  Port=2
  system_flow_in : Inport  Port=3
  buscreator_system_bus_out1 : BusCreator  Inputs=2
  ctrl : Subsystem
  memoryctrl : Memory
  plant : Subsystem
      mask Display: disp('mot4_plant_map_Pelec_funTW_volt_in.slx')
  system_bus_out : Outport
  system_effort_out : Outport  Port=2
  system_flow_out : Outport  Port=3
  wires:
  ctrl/1(system_bus_out) -> [ctrl]  "system_info_bus"
  ctrl/2(local_info_bus_out) -> memoryctrl/1  "ctrl_bus"
  main_info_bus_in/1 -> ctrl/1(main_info_bus_in), plant/1(aInport--1)  "main_info_bus"
  plant/2(outport-plant_bus) -> ctrl/2(local_info_bus_in)  "plant_bus"
  memoryctrl/1 -> plant/2(inport-ctrl_bus-2)  "ctrl_bus"
  plant/1(outport-system_info_bus) -> [plant]  "system_info_bus"
  plant/3(out-effort-7) -> system_effort_out/1  "effort"
  plant/4(out-flow-8) -> system_flow_out/1  "flow"
  system_effort_in/1 -> plant/3(in-effort-2)  "effort"
  system_flow_in/1 -> plant/4(in-flow-3)  "flow"
  buscreator_system_bus_out1/1 -> system_bus_out/1  "system_info_bus"
  [ctrl] -> buscreator_system_bus_out1/1  "ctrl"
  [plant] -> buscreator_system_bus_out1/2  "plant"

== system PowerSystemRef/powerplant/propel ==
  main_info_bus_in : Inport
  system_effort_in : Inport  Port=2
  system_flow_in : Inport  Port=3
  Ground_1 : Ground
  Terminator_1 : Terminator
  plant : Subsystem
      mask Display: disp('propel_plant_uas.slx')
  system_bus_out : Outport
  system_effort_out : Outport  Port=2
  system_flow_out : Outport  Port=3
  wires:
  main_info_bus_in/1 -> plant/1(inport-main_info_bus-1)
  plant/1(outport-system_info_bus) -> [plant]
  plant/3(out-effort-5) -> system_effort_out/1
  plant/4(out-flow-6) -> system_flow_out/1
  system_effort_in/1 -> plant/3(in-effort-4)
  system_flow_in/1 -> plant/4(in-flow-5)
  [plant] -> system_bus_out/1  "plant"
  Ground_1/1 -> plant/2(aInport--2)
  plant/2(aOutport--2) -> Terminator_1/1

== system PowerSystemRef/powerplant/propel2 ==
  main_info_bus_in : Inport
  system_effort_in : Inport  Port=2
  system_flow_in : Inport  Port=3
  Ground_1 : Ground
  Terminator_1 : Terminator
  plant : Subsystem
      mask Display: disp('propel2_plant_uas.slx')
  system_bus_out : Outport
  system_effort_out : Outport  Port=2
  system_flow_out : Outport  Port=3
  wires:
  main_info_bus_in/1 -> plant/1(inport-main_info_bus-1)
  plant/1(outport-system_info_bus) -> [plant]
  plant/3(out-effort-5) -> system_effort_out/1
  plant/4(out-flow-6) -> system_flow_out/1
  system_effort_in/1 -> plant/3(in-effort-4)
  system_flow_in/1 -> plant/4(in-flow-5)
  [plant] -> system_bus_out/1  "plant"
  Ground_1/1 -> plant/2(aInport--2)
  plant/2(aOutport--2) -> Terminator_1/1

== system PowerSystemRef/powerplant/propel3 ==
  main_info_bus_in : Inport
  system_effort_in : Inport  Port=2
  system_flow_in : Inport  Port=3
  Ground_1 : Ground
  Terminator_1 : Terminator
  plant : Subsystem
      mask Display: disp('propel3_plant_uas.slx')
  system_bus_out : Outport
  system_effort_out : Outport  Port=2
  system_flow_out : Outport  Port=3
  wires:
  main_info_bus_in/1 -> plant/1(inport-main_info_bus-1)
  plant/1(outport-system_info_bus) -> [plant]
  plant/3(out-effort-5) -> system_effort_out/1
  plant/4(out-flow-6) -> system_flow_out/1
  system_effort_in/1 -> plant/3(in-effort-4)
  system_flow_in/1 -> plant/4(in-flow-5)
  [plant] -> system_bus_out/1  "plant"
  Ground_1/1 -> plant/2(aInport--2)
  plant/2(aOutport--2) -> Terminator_1/1

== system PowerSystemRef/powerplant/propel4 ==
  main_info_bus_in : Inport
  system_effort_in : Inport  Port=2
  system_flow_in : Inport  Port=3
  Ground_1 : Ground
  Terminator_1 : Terminator
  plant : Subsystem
      mask Display: disp('propel4_plant_uas.slx')
  system_bus_out : Outport
  system_effort_out : Outport  Port=2
  system_flow_out : Outport  Port=3
  wires:
  main_info_bus_in/1 -> plant/1(inport-main_info_bus-1)
  plant/1(outport-system_info_bus) -> [plant]
  plant/3(out-effort-5) -> system_effort_out/1
  plant/4(out-flow-6) -> system_flow_out/1
  system_effort_in/1 -> plant/3(in-effort-4)
  system_flow_in/1 -> plant/4(in-flow-5)
  [plant] -> system_bus_out/1  "plant"
  Ground_1/1 -> plant/2(aInport--2)
  plant/2(aOutport--2) -> Terminator_1/1

== system PowerSystemRef/powerplant/tc ==
  main_info_bus_in : Inport
  system_effort_in : Inport  Port=2
  system_flow_in : Inport  Port=3
  Ground_1 : Ground
  Terminator_1 : Terminator
  plant : Subsystem
      mask Display: disp('tc_plant_map_trqloss_funTW.slx')
  system_bus_out : Outport
  system_effort_out : Outport  Port=2
  system_flow_out : Outport  Port=3
  wires:
  main_info_bus_in/1 -> plant/1(aInport--1)
  plant/1(outport-system_info_bus) -> [plant]
  plant/3(out-effort-7) -> system_effort_out/1
  plant/4(out-flow-8) -> system_flow_out/1
  system_effort_in/1 -> plant/3(in-effort-1)
  system_flow_in/1 -> plant/4(in-flow-2)
  [plant] -> system_bus_out/1  "plant"
  Ground_1/1 -> plant/2(aInport--2)
  plant/2(aOutport--2) -> Terminator_1/1

== system PowerSystemRef/powerplant/tc2 ==
  main_info_bus_in : Inport
  system_effort_in : Inport  Port=2
  system_flow_in : Inport  Port=3
  Ground_1 : Ground
  Terminator_1 : Terminator
  plant : Subsystem
      mask Display: disp('tc2_plant_map_trqloss_funTW.slx')
  system_bus_out : Outport
  system_effort_out : Outport  Port=2
  system_flow_out : Outport  Port=3
  wires:
  main_info_bus_in/1 -> plant/1(aInport--1)
  plant/1(outport-system_info_bus) -> [plant]
  plant/3(out-effort-7) -> system_effort_out/1
  plant/4(out-flow-8) -> system_flow_out/1
  system_effort_in/1 -> plant/3(in-effort-1)
  system_flow_in/1 -> plant/4(in-flow-2)
  [plant] -> system_bus_out/1  "plant"
  Ground_1/1 -> plant/2(aInport--2)
  plant/2(aOutport--2) -> Terminator_1/1

== system PowerSystemRef/powerplant/tc3 ==
  main_info_bus_in : Inport
  system_effort_in : Inport  Port=2
  system_flow_in : Inport  Port=3
  Ground_1 : Ground
  Terminator_1 : Terminator
  plant : Subsystem
      mask Display: disp('tc3_plant_map_trqloss_funTW.slx')
  system_bus_out : Outport
  system_effort_out : Outport  Port=2
  system_flow_out : Outport  Port=3
  wires:
  main_info_bus_in/1 -> plant/1(aInport--1)
  plant/1(outport-system_info_bus) -> [plant]
  plant/3(out-effort-7) -> system_effort_out/1
  plant/4(out-flow-8) -> system_flow_out/1
  system_effort_in/1 -> plant/3(in-effort-1)
  system_flow_in/1 -> plant/4(in-flow-2)
  [plant] -> system_bus_out/1  "plant"
  Ground_1/1 -> plant/2(aInport--2)
  plant/2(aOutport--2) -> Terminator_1/1

== system PowerSystemRef/powerplant/tc4 ==
  main_info_bus_in : Inport
  system_effort_in : Inport  Port=2
  system_flow_in : Inport  Port=3
  Ground_1 : Ground
  Terminator_1 : Terminator
  plant : Subsystem
      mask Display: disp('tc4_plant_map_trqloss_funTW.slx')
  system_bus_out : Outport
  system_effort_out : Outport  Port=2
  system_flow_out : Outport  Port=3
  wires:
  main_info_bus_in/1 -> plant/1(aInport--1)
  plant/1(outport-system_info_bus) -> [plant]
  plant/3(out-effort-7) -> system_effort_out/1
  plant/4(out-flow-8) -> system_flow_out/1
  system_effort_in/1 -> plant/3(in-effort-1)
  system_flow_in/1 -> plant/4(in-flow-2)
  [plant] -> system_bus_out/1  "plant"
  Ground_1/1 -> plant/2(aInport--2)
  plant/2(aOutport--2) -> Terminator_1/1

== system PowerSystemRef/propel/plant ==
  inport-main_info_bus-1 : Inport
  aInport--2 : Inport  Port=2
  in-effort-4 : Inport  Port=3
  in-flow-5 : Inport  Port=4
  Ground_1 : Ground
  Terminator_1 : Terminator
  parameter_out : Subsystem
  parameter_selection : Subsystem
  propel_plant_uas : Subsystem
  outport-system_info_bus : Outport
  aOutport--2 : Outport  Port=2
  out-effort-5 : Outport  Port=3
  out-flow-6 : Outport  Port=4
  wires:
  inport-main_info_bus-1/1 -> parameter_selection/1(inport-main_info_bus-1)
  parameter_out/1(outport-system_info_bus) -> outport-system_info_bus/1
  propel_plant_uas/1(propel_plant_speed_simu) -> parameter_out/1(inport-propel_plant_speed_simu)
  propel_plant_uas/2(propel_plant_pwr_in_simu) -> parameter_out/2(inport-propel_plant_pwr_in_simu)
  propel_plant_uas/3(propel_plant_pwr_out_simu) -> parameter_out/3(inport-propel_plant_pwr_out_simu)
  propel_plant_uas/4(propel_plant_thrust_simu) -> parameter_out/4(inport-propel_plant_thrust_simu)
  parameter_selection/1(outport-env_plant_density_simu-1) -> propel_plant_uas/1(env_plant_density_simu)
  parameter_selection/2(outport-tc_plant_inertia_out_simu-2) -> propel_plant_uas/2(tc_plant_inertia_out_simu)
  parameter_selection/3(outport-eqnmotion_plant_linvel_simu-3) -> propel_plant_uas/3(eqnmotion_plant_linvel_simu)
  in-effort-4/1 -> propel_plant_uas/4(tc_plant_trq_out_simu)
  in-flow-5/1 -> propel_plant_uas/5(flow-in)
  propel_plant_uas/5(propel_plant_effort) -> out-effort-5/1
  propel_plant_uas/6(propel_plant_speed_out_simu) -> out-flow-6/1
  aInport--2/1 -> Terminator_1/1
  Ground_1/1 -> aOutport--2/1

== system PowerSystemRef/tc/plant ==
  aInport--1 : Inport
  aInport--2 : Inport  Port=2
  in-effort-1 : Inport  Port=3
  in-flow-2 : Inport  Port=4
  Ground_1 : Ground
  Terminator_1 : Terminator
  Terminator_2 : Terminator
  parameter_out : Subsystem
  parameter_selection : Subsystem
  tc_plant_map_trqloss_funTW : Subsystem
  outport-system_info_bus : Outport
  aOutport--2 : Outport  Port=2
  out-effort-7 : Outport  Port=3
  out-flow-8 : Outport  Port=4
  wires:
  parameter_out/1(outport-system_info_bus) -> outport-system_info_bus/1
  tc_plant_map_trqloss_funTW/1(tc_plant_trq_in_simu) -> parameter_out/1(inport-tc_plant_trq_in_simu)
  tc_plant_map_trqloss_funTW/2(tc_plant_trq_out_simu) -> parameter_out/2(inport-tc_plant_trq_out_simu)
  tc_plant_map_trqloss_funTW/3(tc_plant_spd_in_simu) -> parameter_out/3(inport-tc_plant_spd_in_simu)
  tc_plant_map_trqloss_funTW/4(tc_plant_spd_out_simu) -> parameter_out/4(inport-tc_plant_spd_out_simu)
  tc_plant_map_trqloss_funTW/5(tc_plant_inertia_in_simu) -> parameter_out/5(inport-tc_plant_inertia_in_simu)
  tc_plant_map_trqloss_funTW/6(tc_plant_inertia_out_simu) -> parameter_out/6(inport-tc_plant_inertia_out_simu)
  in-effort-1/1 -> tc_plant_map_trqloss_funTW/1(tc_trq_in tc_inertia_in)
  in-flow-2/1 -> tc_plant_map_trqloss_funTW/2(tc_spd_out)
  tc_plant_map_trqloss_funTW/7(tc_trq_out) -> out-effort-7/1
  tc_plant_map_trqloss_funTW/8(tc_spd_in) -> out-flow-8/1
  aInport--1/1 -> Terminator_1/1
  aInport--2/1 -> Terminator_2/1
  Ground_1/1 -> aOutport--2/1

== system PowerSystemRef/accelec/plant/accelec_plant_const_pwrloss_volt_in_nokey ==
  drv_key_on_dmd_simu : Inport
  accelec_volt_in : Inport  Port=2
  accelec_curr_out : Inport  Port=3
  Electrical Power : Constant  Value=accelec.plant.init.pwr
  Product : Product  Inputs=*/  InputSameDT=on  SaturateOnIntegerOverflow=on  OutDataTypeStr=Inherit: Same as first input
  Sum : Sum  InputSameDT=on  SaturateOnIntegerOverflow=on  OutDataTypeStr=Inherit: Same as first input
  Sum1 : Sum  InputSameDT=on  SaturateOnIntegerOverflow=on  OutDataTypeStr=Inherit: Same as first input
  Terminator : Terminator
  eps : Constant  Value=eps
  goto_accelec_plant_curr_simu : Goto  Commented=on  GotoTag=accelec_plant_curr_simu
  accelec_plant_volt_in_simu : Outport  VectorParamsAs1DForOutWhenUnconnected=off
  accelec_plant_pwr_simu : Outport  Port=2  VectorParamsAs1DForOutWhenUnconnected=off
  accelec_plant_curr_in_simu : Outport  Port=3  VectorParamsAs1DForOutWhenUnconnected=off
  accelec_plant_volt_out_simu : Outport  Port=4  VectorParamsAs1DForOutWhenUnconnected=off
  accelec_plant_curr_out_simu : Outport  Port=5  VectorParamsAs1DForOutWhenUnconnected=off
  accelec_volt_out : Outport  Port=6  VectorParamsAs1DForOutWhenUnconnected=off
  accelec_curr_in : Outport  Port=7  VectorParamsAs1DForOutWhenUnconnected=off
  wires:
  drv_key_on_dmd_simu/1 -> Terminator/1
  Electrical Power/1 -> Product/1, [accelec_plant_pwr_simu]
  [accelec_plant_volt_out_simu] -> accelec_plant_volt_out_simu/1  "accelec_plant_volt_out_simu"
  [accelec_plant_curr_out_simu] -> accelec_plant_curr_out_simu/1  "accelec_plant_curr_out_simu"
  [accelec_plant_curr_in_simu] -> accelec_plant_curr_in_simu/1  "accelec_plant_curr_in_simu"
  Sum1/1 -> Product/2
  Sum/1 -> accelec_curr_in/1, [accelec_plant_curr_in_simu]
  accelec_curr_out/1 -> Sum/2, [accelec_plant_curr_out_simu]
  Product/1 -> Sum/1, goto_accelec_plant_curr_simu/1
  eps/1 -> Sum1/2
  [accelec_plant_volt_in_simu] -> accelec_plant_volt_in_simu/1  "accelec_plant_volt_in_simu"
  accelec_volt_in/1 -> accelec_volt_out/1, [accelec_plant_volt_out_simu], [accelec_plant_volt_in_simu], Sum1/1
  [accelec_plant_pwr_simu] -> accelec_plant_pwr_simu/1  "accelec_plant_pwr_simu"

== system PowerSystemRef/accelec/plant/parameter_out ==
  inport-accelec_plant_volt_in_simu : Inport
  inport-accelec_plant_pwr_simu : Inport  Port=2
  inport-accelec_plant_curr_in_simu : Inport  Port=3
  inport-accelec_plant_volt_out_simu : Inport  Port=4
  inport-accelec_plant_curr_out_simu : Inport  Port=5
  Ground_1 : Ground
  Toworkspace-accelec_plant_curr_in_simu : ToWorkspace  VariableName=accelec_plant_curr_in_simu  SampleTime=pxf_diagram_options.workspace_sample_time
      settings: Decimation=pxf_diagram_options.decimation
  Toworkspace-accelec_plant_curr_out_simu : ToWorkspace  VariableName=accelec_plant_curr_out_simu  SampleTime=pxf_diagram_options.workspace_sample_time
      settings: Decimation=pxf_diagram_options.decimation
  Toworkspace-accelec_plant_pwr_simu : ToWorkspace  VariableName=accelec_plant_pwr_simu  SampleTime=pxf_diagram_options.workspace_sample_time
      settings: Decimation=pxf_diagram_options.decimation
  Toworkspace-accelec_plant_volt_in_simu : ToWorkspace  VariableName=accelec_plant_volt_in_simu  SampleTime=pxf_diagram_options.workspace_sample_time
      settings: Decimation=pxf_diagram_options.decimation
  Toworkspace-accelec_plant_volt_out_simu : ToWorkspace  VariableName=accelec_plant_volt_out_simu  SampleTime=pxf_diagram_options.workspace_sample_time
      settings: Decimation=pxf_diagram_options.decimation
  outport-system_info_bus : Outport
  wires:
  inport-accelec_plant_volt_in_simu/1 -> Toworkspace-accelec_plant_volt_in_simu/1
  inport-accelec_plant_pwr_simu/1 -> Toworkspace-accelec_plant_pwr_simu/1
  inport-accelec_plant_curr_in_simu/1 -> Toworkspace-accelec_plant_curr_in_simu/1
  inport-accelec_plant_volt_out_simu/1 -> Toworkspace-accelec_plant_volt_out_simu/1
  inport-accelec_plant_curr_out_simu/1 -> Toworkspace-accelec_plant_curr_out_simu/1
  Ground_1/1 -> outport-system_info_bus/1

== system PowerSystemRef/accelec/plant/parameter_selection ==

== system PowerSystemRef/ess (battery)/ctrl/ess_ctrl_pngv_map_anl_PI_cstr ==
  ess_volt_out : Inport
  ess_curr_out : Inport  Port=2
  ess_soc : Inport  Port=3
  Demux : Demux  Outputs=3
  Demux1 : Demux  Outputs=3
  PI controller for maximal charge power and current1 : Subsystem
  PI controller for maximal discharge power and current1 : Subsystem
  mux1 : Mux  Inputs=3
  ess_ctrl_pwr_max_pro_simu : Outport
  ess_ctrl_pwr_max_reg_simu : Outport  Port=2
  ess_ctrl_curr_max_pro_simu : Outport  Port=3
  ess_ctrl_curr_max_reg_simu : Outport  Port=4
  wires:
  ess_soc/1 -> mux1/3  "ess_plant_soc_simu"
  ess_curr_out/1 -> mux1/2  "ess_plant_curr_out_simu"
  Demux1/3 -> PI controller for maximal charge power and current1/3(SOC)
  Demux1/2 -> PI controller for maximal charge power and current1/2(ess curr)
  Demux1/1 -> PI controller for maximal charge power and current1/1(ess voltage)
  Demux/3 -> PI controller for maximal discharge power and current1/3(SOC)
  Demux/2 -> PI controller for maximal discharge power and current1/2(ess curr)
  Demux/1 -> PI controller for maximal discharge power and current1/1(ess voltage)
  PI controller for maximal charge power and current1/1(Pwr_max_reg) -> [ess_ctrl_pwr_max_reg_simu]
  PI controller for maximal discharge power and current1/2(Pwr_max_prop) -> [ess_ctrl_pwr_max_pro_simu]
  mux1/1 -> Demux1/1, Demux/1
  ess_volt_out/1 -> mux1/1  "ess_plant_volt_out_simu"
  PI controller for maximal charge power and current1/2(Curr_max_reg) -> [ess_ctrl_curr_max_reg_simu]
  PI controller for maximal discharge power and current1/1(Curr_max_prop) -> [ess_ctrl_curr_max_pro_simu]
  [ess_ctrl_curr_max_reg_simu] -> ess_ctrl_curr_max_reg_simu/1  "ess_ctrl_curr_max_reg_simu"
  [ess_ctrl_curr_max_pro_simu] -> ess_ctrl_curr_max_pro_simu/1  "ess_ctrl_curr_max_pro_simu"
  [ess_ctrl_pwr_max_pro_simu] -> ess_ctrl_pwr_max_pro_simu/1  "ess_ctrl_pwr_max_pro_simu"
  [ess_ctrl_pwr_max_reg_simu] -> ess_ctrl_pwr_max_reg_simu/1  "ess_ctrl_pwr_max_reg_simu"

== system PowerSystemRef/ess (battery)/ctrl/parameter_out ==
  inport-ess_ctrl_pwr_max_pro_simu : Inport
  inport-ess_ctrl_pwr_max_reg_simu : Inport  Port=2
  inport-ess_ctrl_curr_max_pro_simu : Inport  Port=3
  inport-ess_ctrl_curr_max_reg_simu : Inport  Port=4
  Ground_1 : Ground
  Toworkspace-ess_ctrl_curr_max_pro_simu : ToWorkspace  VariableName=ess_ctrl_curr_max_pro_simu  SampleTime=pxf_diagram_options.workspace_sample_time
      settings: Decimation=pxf_diagram_options.decimation
  Toworkspace-ess_ctrl_curr_max_reg_simu : ToWorkspace  VariableName=ess_ctrl_curr_max_reg_simu  SampleTime=pxf_diagram_options.workspace_sample_time
      settings: Decimation=pxf_diagram_options.decimation
  Toworkspace-ess_ctrl_pwr_max_pro_simu : ToWorkspace  VariableName=ess_ctrl_pwr_max_pro_simu  SampleTime=pxf_diagram_options.workspace_sample_time
      settings: Decimation=pxf_diagram_options.decimation
  Toworkspace-ess_ctrl_pwr_max_reg_simu : ToWorkspace  VariableName=ess_ctrl_pwr_max_reg_simu  SampleTime=pxf_diagram_options.workspace_sample_time
      settings: Decimation=pxf_diagram_options.decimation
  create_system_info_bus : BusCreator  Inputs=1
  outport-system_info_bus : Outport
  outport-ctrl_bus : Outport  Port=2
  wires:
  create_system_info_bus/1 -> outport-system_info_bus/1
  inport-ess_ctrl_pwr_max_pro_simu/1 -> create_system_info_bus/1, Toworkspace-ess_ctrl_pwr_max_pro_simu/1  "ess_ctrl_pwr_max_pro_simu"
  inport-ess_ctrl_pwr_max_reg_simu/1 -> Toworkspace-ess_ctrl_pwr_max_reg_simu/1
  inport-ess_ctrl_curr_max_pro_simu/1 -> Toworkspace-ess_ctrl_curr_max_pro_simu/1
  inport-ess_ctrl_curr_max_reg_simu/1 -> Toworkspace-ess_ctrl_curr_max_reg_simu/1
  Ground_1/1 -> outport-ctrl_bus/1

== system PowerSystemRef/ess (battery)/ctrl/parameter_selection ==
  inport-main_info_bus-1 : Inport
  select_main_info_bus : BusSelector  OutputSignals=ess.plant.ess_plant_volt_out_simu,ess.plant.ess_plant_curr_out_simu,ess.plant.ess_plant_soc_simu
  outport-ess_plant_volt_out_simu-1 : Outport
  outport-ess_plant_curr_out_simu-2 : Outport  Port=2
  outport-ess_plant_soc_simu-3 : Outport  Port=3
  wires:
  inport-main_info_bus-1/1 -> select_main_info_bus/1
  select_main_info_bus/1 -> outport-ess_plant_volt_out_simu-1/1  "<ess_plant_volt_out_simu>"
  select_main_info_bus/2 -> outport-ess_plant_curr_out_simu-2/1  "<ess_plant_curr_out_simu>"
  select_main_info_bus/3 -> outport-ess_plant_soc_simu-3/1  "<ess_plant_soc_simu>"
